simulink model "mainmodel"  (R2020a)
settings: Solver=VariableStepAuto  StartTime=0.0  StopTime=10.0  RelTol=1e-3
settings Model: Creator=Bhanu  LastModifiedBy=Bhanu

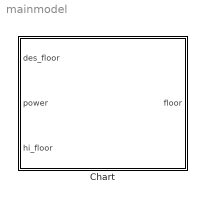
== system mainmodel ==
  Chart : Stateflow chart  TreatAsAtomicUnit=on

== stateflow chart mainmodel/Chart ==
  state powerOn
    state Idle
      state Close
      state Open
        en: delay = delay+1;
      (default) -> Close
      Close -> Open : obj_detect [floor == des_floor]
      Open -> Close [order 1] : [delay == 3]/{delay == 0}
      Open -> Open [order 2] : [delay < 3]
    state Up
      en: floor = floor + 1;
    state highestFloor
      en: floor = hi_floor;
    state Down1
      en: floor = 0;
    state Down
      en: floor = floor -1;
    (default) -> Idle
    Up -> Idle [order 1] : [floor == des_floor]
    Down -> Idle [order 1] : [floor == des_floor]
    Idle -> Down [order 2] : [floor > des_floor]
    Idle -> Up [order 1] : [floor < des_floor]
    highestFloor -> Idle
    Up -> highestFloor [order 3] : [des_floor > hi_floor]
    Down -> Down1 [order 3] : [des_floor < 0]
    Down -> Down [order 2] : [floor > des_floor]
    Up -> Up [order 2] : [floor < des_floor]
  state powerOff
    en: floor = 0;
  (default) -> powerOff
  powerOff -> powerOn : [power == 1]
  powerOn -> powerOff : [power == 0]
  data: des_floor input; delay local; power input; hi_floor input; floor output
  events: obj_detect local FUNCTION_CALL_EVENT
